simulink model "sw11"  (Simulink 7.9)
settings: Solver=ode4  StartTime=0.0  StopTime=20.0  FixedStep=5e-3  RelTol=1e-6
undefined symbols (not defined in the file): a, c, g, m
settings Model: Creator=Daniel  LastModifiedBy=Daniel
settings DataIOCC: LimitDataPoints=off

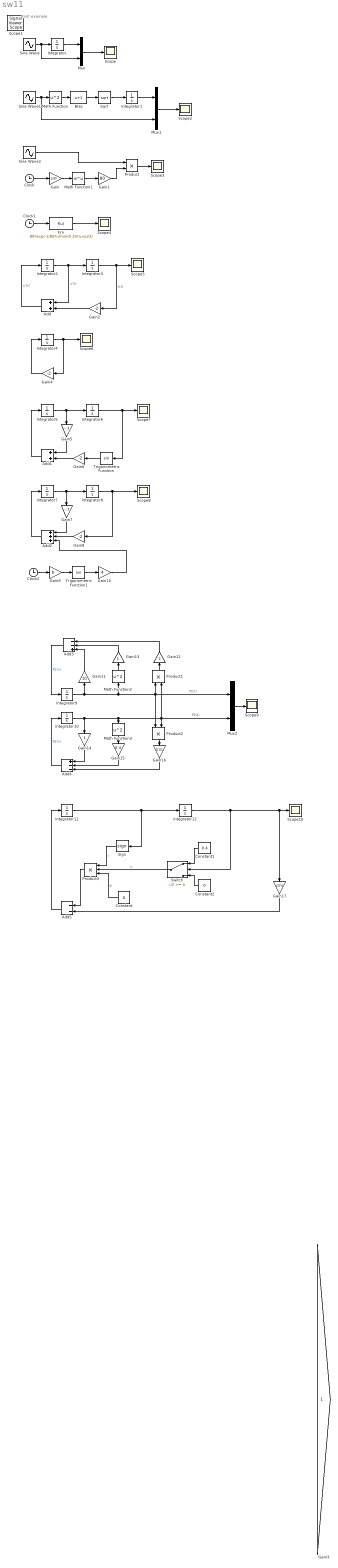
== system sw11 ==
  note: First example
  Add : Sum
  Add1 : Sum
  Add2 : Sum  Inputs=+++
  Add3 : Sum  Inputs=--+
  Add4 : Sum  Inputs=+--
  Add5 : Sum  Inputs=--
  Bias : Bias  Bias=1
  Clock : Clock
  Clock1 : Clock
  Clock2 : Clock
  Constant : Constant  Value=g
  Constant1 : Constant  Value=0.4
  Constant2 : Constant  Value=0
  Fcn : Fcn  Expr=80*exp(-1/80*u)*sin(0.25*u+pi/3)
  Gain : Gain  Gain=-1/80
  Gain1 : Gain  Gain=80
  Gain10 : Gain  Gain=4
  Gain11 : Gain  Gain=10
  Gain12 : Gain  Gain=2
  Gain13 : Gain
  Gain14 : Gain
  Gain15 : Gain  Gain=0.4
  Gain16 : Gain  Gain=0.01
  Gain17 : Gain  Gain=c/m
  Gain{2,4,6,8} (4 alike) : Gain  Gain=-2
  Gain3 : Gain
  Gain5 : Gain  Gain=-.7
  Gain7 : Gain  Gain=-.7
  Gain9 : Gain  Gain=6
  Integrator{,1,5,7..8,11} (6 alike) : Integrator
  Integrator10 : Integrator  InitialCondition=10
  Integrator12 : Integrator  InitialCondition=4*a
  Integrator2 : Integrator  InitialCondition=2
  Integrator3 : Integrator  InitialCondition=1
  Integrator4 : Integrator  InitialCondition=1
  Integrator6 : Integrator  InitialCondition=pi/4
  Integrator9 : Integrator  InitialCondition=5
  Math Function : Math  Operator=square  SaturateOnIntegerOverflow=on
  Math Function1 : Math  SaturateOnIntegerOverflow=on
  Math Function2 : Math  Operator=square  SaturateOnIntegerOverflow=on
  Math Function3 : Math  Operator=square  SaturateOnIntegerOverflow=on
  Mux : Mux  Inputs=2
  Mux1 : Mux  Inputs=2
  Mux2 : Mux  Inputs=2
  Product : Product  RndMeth=Zero
  Product1 : Product  RndMeth=Zero
  Product2 : Product  RndMeth=Zero
  Product3 : Product  Inputs=3  RndMeth=Zero
  Scope{,2..10} (10 alike) : Scope
      Scope10 settings: SaveName=ScopeData9
      Scope3 settings: SaveName=ScopeData2
      Scope4 settings: SaveName=ScopeData3
      Scope5 settings: SaveName=ScopeData4
      Scope6 settings: SaveName=ScopeData5
      Scope7 settings: SaveName=ScopeData6
      Scope8 settings: SaveName=ScopeData7
      Scope9 settings: SaveName=ScopeData8
  Sign : Signum
  Sine Wave : Sin  Frequency=3  SampleTime=0
  Sine Wave1 : Sin  Frequency=0.8  SampleTime=0
  Sine Wave2 : Sin  Frequency=0.25  Phase=pi/3  SampleTime=0
  Sqrt : Sqrt  SaturateOnIntegerOverflow=on
  Switch : Switch  Threshold=a
  Trigonometric Function : Trigonometry
  Trigonometric Function1 : Trigonometry
  Scope1 : SignalViewerScope  IOType=viewer  RefreshTime=0.035000
  wires:
  Sine Wave/1 -> Integrator/1, Mux/2
  Integrator/1 -> Mux/1
  Mux/1 -> Scope/1
  Sine Wave1/1 -> Mux1/2, Math Function/1
  Integrator1/1 -> Mux1/1
  Mux1/1 -> Scope2/1
  Sqrt/1 -> Integrator1/1
  Bias/1 -> Sqrt/1
  Math Function/1 -> Bias/1
  Clock/1 -> Gain/1
  Gain/1 -> Math Function1/1
  Math Function1/1 -> Gain1/1
  Sine Wave2/1 -> Product/1
  Gain1/1 -> Product/2
  Product/1 -> Scope3/1
  Clock1/1 -> Fcn/1
  Fcn/1 -> Scope4/1
  Integrator2/1 -> Integrator3/1, Add/1  "x'(t)"
  Gain2/1 -> Add/2
  Add/1 -> Integrator2/1  "x''(t)"
  Integrator3/1 -> Gain2/1, Scope5/1  "x(t)"
  Gain4/1 -> Integrator4/1
  Integrator4/1 -> Gain4/1, Scope6/1
  Add1/1 -> Integrator5/1
  Integrator5/1 -> Integrator6/1, Gain5/1
  Gain5/1 -> Add1/1
  Gain6/1 -> Add1/2
  Trigonometric Function/1 -> Gain6/1
  Integrator6/1 -> Trigonometric Function/1, Scope7/1
  Add2/1 -> Integrator7/1
  Integrator7/1 -> Gain7/1, Integrator8/1
  Gain7/1 -> Add2/1
  Gain8/1 -> Add2/2
  Integrator8/1 -> Gain8/1, Scope8/1
  Trigonometric Function1/1 -> Gain10/1
  Clock2/1 -> Gain9/1
  Gain9/1 -> Trigonometric Function1/1
  Gain10/1 -> Add2/3
  Add3/1 -> Integrator9/1  "P1'(t)"
  Add4/1 -> Integrator10/1  "P2'(t)"
  Integrator9/1 -> Gain11/1, Math Function2/1, Product1/1, Product2/1, Mux2/1  "P1(t)"
  Integrator10/1 -> Product1/2, Product2/2, Mux2/2, Math Function3/1, Gain14/1  "P2(t)"
  Gain11/1 -> Add3/3
  Math Function2/1 -> Gain13/1
  Product1/1 -> Gain12/1
  Gain12/1 -> Add3/1
  Gain13/1 -> Add3/2
  Gain14/1 -> Add4/1
  Math Function3/1 -> Gain15/1
  Gain15/1 -> Add4/2
  Product2/1 -> Gain16/1
  Gain16/1 -> Add4/3
  Mux2/1 -> Scope9/1
  Add5/1 -> Integrator11/1
  Integrator11/1 -> Integrator12/1, Sign/1
  Integrator12/1 -> Scope10/1, Gain17/1, Switch/2
  Gain17/1 -> Add5/2
  Sign/1 -> Product3/1  "r"
  Constant/1 -> Product3/3  "g"
  Product3/1 -> Add5/1
  Switch/1 -> Product3/2  "u"
  Constant1/1 -> Switch/1
  Constant2/1 -> Switch/3
